simulink library "hdlsllibUNLOCKED"  (R2019a)
settings: Solver=ode45  StartTime=0.0  StopTime=10.0  RelTol=1e-3  EnableMultiTasking=on
values from neighbouring files (symbols this model uses):
  freerun = strcmp(get_param(blk, 'CountType'), 'Free running')    [hdlblkmask_counter.m]
  maxval_sc = countrange(2)    [hdlblkmask_counter.m]
  samptime = -1    [hdlblkmask_counter.m]
undefined symbols (not defined in the file or in its folder): a, b, c, Dialog, DiscIntNeverNeededParam, Floor, HDLStatusEnum, jsin, magnitude, message, Newton, NumBits1, NumBits2, Raphson, Slope1, Slope2
libraries: simulink x70, $bdroot x5, hdlmdlgenlib x1, hdlsllib_helper x1
(part 1 of 3)
settings Model: Creator=The MathWorks, Inc kinda  LastModifiedBy=Bailey
settings DataIOCC: LimitDataPoints=on  SaveFormat=Array  ReturnWorkspaceOutputs=off
settings OptimizationCC: LifeSpan=inf
settings DebuggingCC: UnderspecifiedInitializationDetection=Classic  MergeDetectMultiDrivingBlocksExec=none  SolverPrmCheckMsg=warning  AllowSymbolicDim=off  PregeneratedLibrarySubsystemCodeDiagnostic=none  SFUnexpectedBacktrackingDiag=warning  SFNoUnconditionalDefaultTransitionDiag=warning  SFExecutionAtInitializationDiag=none  ArithmeticOperatorsInVariantConditions=warning
settings HardwareCC: ProdBitPerPointer=32  ProdBitPerSizeT=32  ProdBitPerPtrDiffT=32  ProdLargestAtomicFloat=None  ProdIntDivRoundTo=Undefined  ProdEndianess=Unspecified  ProdWordSize=32  ProdHWDeviceType=32-bit Generic
settings ModelReferenceCC: PropagateSignalLabelsOutOfModel=off
settings SFSimCC: SimUseLocalCustomCode=off
settings RTWCC: RTWUseLocalCustomCode=off
settings CodeAppCC: StateflowObjectComments=on
settings GRTTargetCC: TargetLangStandard=C89/C90 (ANSI)  GeneratePreprocessorConditionals=Disable all
settings ConfigComp: CovScope=ReferencedModels  CovMetricSettings=dw  CovHtmlReporting=on  CovSaveCumulativeToWorkspaceVar=on  CovSaveSingleToWorkspaceVar=on  CovShowResultsExplorer=off  CovExternalEMLEnable=off  CovSFcnEnable=off

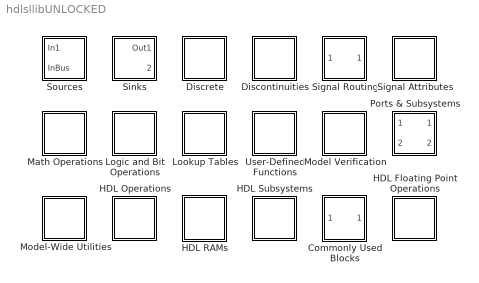
== system hdlsllibUNLOCKED ==
  Commonly Used Blocks : Subsystem
      mask Display: image('commonly_used.bmp')
  Discontinuities : Subsystem
      mask Display: image('nonlinear.bmp')
  Discrete : Subsystem
      mask Display: image('discrete.bmp')
  HDL Subsystems : Subsystem
      mask Display:
      | image('blank_block.bmp')
      | color('darkBlue')
      | fprintf('HDL\nSubsys\n')
  HDL Floating Point Operations : Subsystem
      mask Display:
      | image('blank_block.bmp')
      | color('darkBlue')
      | fprintf(' HDL\nNFP')
  HDL Operations : Subsystem
      mask Display:
      | image('blank_block.bmp')
      | color('darkBlue')
      | fprintf(' HDL\nOPS')
  HDL RAMs : Subsystem
      mask Display:
      | image('blank_block.bmp')
      | color('darkBlue')
      | fprintf(' HDL\nRAMs')
  Logic and Bit Operations : Subsystem
      mask Display: image('logical_bit.bmp')
  Lookup Tables : Subsystem
      mask Display: image('tables.bmp')
  Math Operations : Subsystem
      mask Display: image('math.bmp')
  Model Verification : Subsystem
      mask Display: image('assertion.bmp')
  Model-Wide Utilities : Subsystem
      mask Display:
      | image('blank_block.bmp')
      | color('darkBlue')
      | disp('Misc')
  Ports & Subsystems : Subsystem
      settings: CopyFcn=set_param(gcbh,'LinkStatus','none'); set_param(gcbh,'Mask','off'); set_param(gcbh,'MaskType',''); set_param(gcbh,'MaskDescription',''); set_param(gcbh,'OpenFcn',''); set_param(gcbh,'CopyFcn','')
      mask Display: image('subsystems.bmp')
  Signal Attributes : Subsystem
      mask Display: image('attributes.bmp')
  Signal Routing : Subsystem
      mask Display: image('signals.bmp')
  Sinks : Subsystem
      mask Display: image('sinks.bmp')
  Sources : Subsystem
      mask Display: image('sources.bmp')
  User-Defined Functions : Subsystem
      mask Display: image('functions.bmp')

== system hdlsllibUNLOCKED/Commonly Used Blocks ==
  In1 : Inport
  Constant : Constant
  Data Type Conversion : DataTypeConversion
  Delay : Delay  DelayLength=1  InitialCondition=0
  Demux : Demux  Outputs=2
  Gain : Gain
  Logical Operator : Logic  AllPortsSameDT=off  OutDataTypeStr=boolean
  Mux : Mux  Inputs=2
  Product : Product
  Relational Operator : RelationalOperator  Operator=<=  OutDataTypeStr=boolean  RndMeth=Nearest
  Scope : Scope
  Sum : Sum  Inputs=|++
  Switch : Switch
  Out1 : Outport

== system hdlsllibUNLOCKED/Discontinuities ==
  Backlash : Backlash
  Coulomb & Viscous Friction : simulink/Discontinuities/Coulomb & Viscous Friction  offset=[1 3 2 0]  gain=1
      settings: SourceProductName=Simulink
  Dead Zone : DeadZone  SaturateOnIntegerOverflow=on
  Dead Zone Dynamic : simulink/Discontinuities/Dead Zone Dynamic
      settings: SourceProductName=Simulink  SourceProductBaseCode=SL
  Hit Crossing : HitCross  HitCrossingDirection=rising
  Relay : Relay
  Saturation : Saturate
  Saturation Dynamic : simulink/Discontinuities/Saturation Dynamic  OutMin=[]  OutMax=[]  OutDataTypeStr=Inherit: Same as second input  OutDataType=fixdt(1, 16)  OutScaling=2^-10  DoSatur=off
  Wrap To Zero : simulink/Discontinuities/Wrap To Zero  Threshold=255
      settings: SourceProductName=Simulink  SourceProductBaseCode=SL

== system hdlsllibUNLOCKED/Discrete ==
  Delay : Delay
  Discrete Transfer Fcn : DiscreteTransferFcn
  Discrete FIR Filter : DiscreteFir
  Discrete PID Controller : simulink/Continuous/PID Controller  Controller=PID  Form=Parallel  TimeDomain=Discrete-time  SampleTime=-1  IntegratorMethod=Forward Euler  FilterMethod=Forward Euler  ControllerParametersSource=internal  P=1  I=1  D=0  UseFilter=on  N=100  TunerSelectOption=Transfer Function Based (PID Tuner App)  InitialConditionSource=internal  InitialConditionForIntegrator=0  InitialConditionForFilter=0  DifferentiatorICPrevScaledInput=0  ExternalReset=none  TrackingMode=off  Kt=1  LimitOutput=off  UpperSaturationLimit=inf  LowerSaturationLimit=-inf  LinearizeAsGain=off  AntiWindupMode=none  Kb=1  POutMin=[]  POutMax=[]  IOutMin=[]  IOutMax=[]  DOutMin=[]  DOutMax=[]  NOutMin=[]  NOutMax=[]  SumOutMin=[]  SumOutMax=[]  SaturationOutMin=[]  SaturationOutMax=[]  PParamMin=[]  PParamMax=[]  IParamMin=[]  IParamMax=[]  DParamMin=[]  DParamMax=[]  NParamMin=[]  NParamMax=[]  KbParamMin=[]  KbParamMax=[]  KtParamMin=[]  KtParamMax=[]  KbOutMin=[]  KbOutMax=[]  KtOutMin=[]  KtOutMax=[]  IntegratorOutMin=[]  IntegratorOutMax=[]  FilterOutMin=[]  FilterOutMax=[]  SumI1OutMin=[]  SumI1OutMax=[]  SumI2OutMin=[]  SumI2OutMax=[]  SumI3OutMin=[]  SumI3OutMax=[]  SumI4OutMin=[]  SumI4OutMax=[]  SumDOutMin=[]  SumDOutMax=[]  DifferentiatorOutMin=[]  DifferentiatorOutMax=[]  FilterDiffOutCoefMin=[]  FilterDiffOutCoefMax=[]  ReciprocalOutMin=[]  ReciprocalOutMax=[]  SumDenOutMin=[]  SumDenOutMax=[]  SumNumOutMin=[]  SumNumOutMax=[]  DivideOutMin=[]  DivideOutMax=[]  IntegratorContinuousStateAttributes=''  IntegratorStateMustResolveToSignalObject=off  IntegratorRTWStateStorageClass=Auto  FilterContinuousStateAttributes=''  FilterStateMustResolveToSignalObject=off  FilterRTWStateStorageClass=Auto  ParallelPVariant=InternalParameters  IdealPVariant=Disabled  IVariant=InternalParameters  DVariant=InternalParameters  IntegratorVariant=Discrete  SatVariant=Disabled  AWVariant=Passthrough  PCopyVariant=Disabled  TRVariant=Disabled  FdbkBlocksVariant=Forward  IdealPFdbkVariant=Disabled  SatFdbkVariant=Disabled  DerivativeFilterVariant=ForwardEulerFilter  NVariant=InternalParameters  NCopyVariant=Disabled  FilterICVariant=InternalICsFilter  IntegratorICVariant=InternalICs  ExternalResetVariant=Disabled  TRSumVariant=Passthrough  SumFdbkVariant=Disabled  SumVariant=Sum_PID
  Discrete-Time Integrator : DiscreteIntegrator  SampleTime=-1  ICPrevOutput=DiscIntNeverNeededParam  ICPrevScaledInput=DiscIntNeverNeededParam
  Enabled Delay : Delay  ShowEnablePort=on
      settings: InputPortMap=u0,e6
  Enabled Resettable Delay : Delay  DelayLength=1  ExternalReset=Level  ShowEnablePort=on
      settings: InputPortMap=u0,e6,r5
  Memory : Memory  InheritSampleTime=on
  Resettable Delay : Delay  DelayLength=1  ExternalReset=Level
      settings: InputPortMap=u0,r5
  Tapped Delay : simulink/Discrete/Tapped Delay  vinit=0.0  samptime=-1  NumDelays=4  DelayOrder=Oldest  includeCurrent=off
  Unit Delay : UnitDelay  SampleTime=-1  HasFrameUpgradeWarning=on
  Unit Delay Enabled Synchronous : Subsystem  mask(Unit Delay Enabled Synchronous){InitialCondition=0.0, SampleTime=-1}
      mask prompts: InitialCondition "Simulink:blkprm_prompts:DelayBlkInitCond"; SampleTime "Simulink:blkprm_prompts:AllBlksSampleTime"
      mask help:
      | Normally, the output is the signal u delayed by one sample period.
      | When the enable signal is false, the block is disabled, and the state and output values do not change. The enable action only supports scalar inputs. Scalar expansion is used for the enable action when the signal u is a vector.
      mask Help: helpview([docroot '/simulink/helptargets.map'],'HDL_Unit_Delay_Enabled_Synchronous');
      mask TypeOptions InitialCondition: Unit Delay Enabled/Enabled Delay/InitialCondition
      mask TypeOptions SampleTime: Unit Delay Enabled/Enabled Delay/SampleTime
      mask DialogControl InitialCondition Prompt: Initial condition:
      mask DialogControl SampleTime Prompt: Sample time (-1 for inherited):
      mask Display: dpoly([0 1],[1 0],'z');
  Unit Delay Enabled Resettable Synchronous : Subsystem  mask(Unit Delay Enabled Resettable Synchronous){InitialCondition=0.0, SampleTime=-1}
      mask prompts: InitialCondition "Simulink:blkprm_prompts:DelayBlkInitCond"; SampleTime "Simulink:blkprm_prompts:AllBlksSampleTime"
      mask help:
      | Normally, the output is the signal u delayed by one sample period.
      | When the enable signal is false, the block is disabled, and the state and output values do not change. The enable action only supports scalar inputs. Scalar expansion is used for the enable action when the signal u is a vector.
      | When the reset signal R is true, the state and the output are always set equal to the initial condition parameter. This block exhibits hardware-friendly reset behavior. This reset action only supports scalar inputs. Scalar expansion is used for this reset action when the signal u is a vector.
      mask Help: helpview([docroot '/simulink/helptargets.map'],'HDL_Unit_Delay_Enabled_Resettable_Synchronous');
      mask TypeOptions InitialCondition: Unit Delay Enabled Resettable/Enabled Resettable Delay/InitialCondition
      mask TypeOptions SampleTime: Unit Delay Enabled Resettable/Enabled Resettable Delay/SampleTime
      mask DialogControl InitialCondition Prompt: Initial condition:
      mask DialogControl SampleTime Prompt: Sample time (-1 for inherited):
      mask Display: dpoly([0 1],[1 0],'z');
  Unit Delay Resettable Synchronous : Subsystem  mask(Unit Delay Resettable Synchronous){InitialCondition=0.0, SampleTime=-1}
      mask prompts: InitialCondition "Simulink:blkprm_prompts:DelayBlkInitCond"; SampleTime "Simulink:blkprm_prompts:AllBlksSampleTime"
      mask help:
      | Normally, the output is the signal u delayed by one sample period.
      | When the reset signal R is true, the state and the output are always set equal to the initial condition parameter. This block exhibits hardware-friendly reset behavior. This reset action only supports scalar inputs. Scalar expansion is used for this reset action when the signal u is a vector.
      mask Help: helpview([docroot '/simulink/helptargets.map'],'HDL_Unit_Delay_Resettable_Synchronous');
      mask TypeOptions InitialCondition: Unit Delay Resettable/Resettable Delay/InitialCondition
      mask TypeOptions SampleTime: Unit Delay Resettable/Resettable Delay/SampleTime
      mask DialogControl InitialCondition Prompt: Initial condition:
      mask DialogControl SampleTime Prompt: Sample time (-1 for inherited):
      mask Display: dpoly([0 1],[1 0],'z');
  Zero-Order Hold : ZeroOrderHold  SampleTime=-1

== system hdlsllibUNLOCKED/HDL Subsystems ==
  Enabled Synchronous Subsystem : Subsystem  TreatAsAtomicUnit=on  mask(Enabled Synchronous Subsystem){}
      mask help: Simulink:masks:EnabledSynchronousSubsystem_MP
      settings: CopyFcn=set_param(gcbh,'LinkStatus','none'); set_param(gcbh,'Mask','off'); set_param(gcbh,'MaskType',''); set_param(gcbh,'MaskDescription',''); set_param(gcbh,'OpenFcn',''); set_param(gcbh,'CopyFcn','')  OpenFcn=open_system(gcbh,'force')
  Resettable Synchronous Subsystem : Subsystem  TreatAsAtomicUnit=on  mask(Resettable Synchronous Subsystem){}
      mask help: Simulink:masks:ResettableSynchronousSubsystem_MP
      settings: CopyFcn=set_param(gcbh,'LinkStatus','none'); set_param(gcbh,'Mask','off'); set_param(gcbh,'MaskType',''); set_param(gcbh,'MaskDescription',''); set_param(gcbh,'OpenFcn',''); set_param(gcbh,'CopyFcn','')  OpenFcn=open_system(gcbh,'force')
  State Control : StateControl  StateControl=Synchronous
  Synchronous Subsystem : Subsystem  mask(Synchronous Subsystem){}
      mask help: Simulink:masks:SynchronousSubsystem_MP
      settings: CopyFcn=set_param(gcbh,'LinkStatus','none'); set_param(gcbh,'Mask','off'); set_param(gcbh,'MaskType',''); set_param(gcbh,'MaskDescription',''); set_param(gcbh,'OpenFcn',''); set_param(gcbh,'CopyFcn','')  OpenFcn=open_system(gcbh,'force')

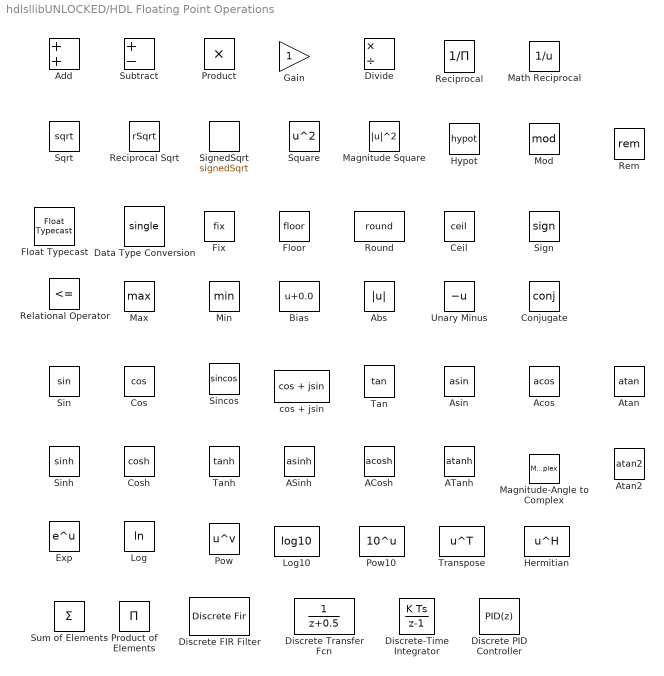
== system hdlsllibUNLOCKED/HDL Floating Point Operations ==
  ACosh : Trigonometry  Operator=acosh
  ASinh : Trigonometry  Operator=asinh
  ATanh : Trigonometry  Operator=atanh
  Abs : Abs
  Acos : Trigonometry  Operator=acos
  Add : Sum
  Asin : Trigonometry  Operator=asin
  Atan : Trigonometry  Operator=atan
  Atan2 : Trigonometry  Operator=atan2
  Bias : Bias  Bias=0.0
  Ceil : Rounding  Operator=ceil
  Conjugate : Math  Operator=conj  RndMeth=Zero  SaturateOnIntegerOverflow=on
  Cos : Trigonometry  Operator=cos
  Cosh : Trigonometry  Operator=cosh
  Data Type Conversion : DataTypeConversion  OutDataTypeStr=single  RndMeth=Nearest
  Discrete Transfer Fcn : DiscreteTransferFcn
  Discrete FIR Filter : DiscreteFir
  Discrete PID Controller : simulink/Continuous/PID Controller  Controller=PID  Form=Parallel  TimeDomain=Discrete-time  SampleTime=-1  IntegratorMethod=Forward Euler  FilterMethod=Forward Euler  ControllerParametersSource=internal  P=1  I=1  D=0  UseFilter=on  N=100  TunerSelectOption=Transfer Function Based (PID Tuner App)  InitialConditionSource=internal  InitialConditionForIntegrator=0  InitialConditionForFilter=0  DifferentiatorICPrevScaledInput=0  ExternalReset=none  TrackingMode=off  Kt=1  LimitOutput=off  UpperSaturationLimit=inf  LowerSaturationLimit=-inf  LinearizeAsGain=off  AntiWindupMode=none  Kb=1  POutMin=[]  POutMax=[]  IOutMin=[]  IOutMax=[]  DOutMin=[]  DOutMax=[]  NOutMin=[]  NOutMax=[]  SumOutMin=[]  SumOutMax=[]  SaturationOutMin=[]  SaturationOutMax=[]  PParamMin=[]  PParamMax=[]  IParamMin=[]  IParamMax=[]  DParamMin=[]  DParamMax=[]  NParamMin=[]  NParamMax=[]  KbParamMin=[]  KbParamMax=[]  KtParamMin=[]  KtParamMax=[]  KbOutMin=[]  KbOutMax=[]  KtOutMin=[]  KtOutMax=[]  IntegratorOutMin=[]  IntegratorOutMax=[]  FilterOutMin=[]  FilterOutMax=[]  SumI1OutMin=[]  SumI1OutMax=[]  SumI2OutMin=[]  SumI2OutMax=[]  SumI3OutMin=[]  SumI3OutMax=[]  SumI4OutMin=[]  SumI4OutMax=[]  SumDOutMin=[]  SumDOutMax=[]  DifferentiatorOutMin=[]  DifferentiatorOutMax=[]  FilterDiffOutCoefMin=[]  FilterDiffOutCoefMax=[]  ReciprocalOutMin=[]  ReciprocalOutMax=[]  SumDenOutMin=[]  SumDenOutMax=[]  SumNumOutMin=[]  SumNumOutMax=[]  DivideOutMin=[]  DivideOutMax=[]  IntegratorContinuousStateAttributes=''  IntegratorStateMustResolveToSignalObject=off  IntegratorRTWStateStorageClass=Auto  FilterContinuousStateAttributes=''  FilterStateMustResolveToSignalObject=off  FilterRTWStateStorageClass=Auto  ParallelPVariant=InternalParameters  IdealPVariant=Disabled  IVariant=InternalParameters  DVariant=InternalParameters  IntegratorVariant=Discrete  SatVariant=Disabled  AWVariant=Passthrough  PCopyVariant=Disabled  TRVariant=Disabled  FdbkBlocksVariant=Forward  IdealPFdbkVariant=Disabled  SatFdbkVariant=Disabled  DerivativeFilterVariant=ForwardEulerFilter  NVariant=InternalParameters  NCopyVariant=Disabled  FilterICVariant=InternalICsFilter  IntegratorICVariant=InternalICs  ExternalResetVariant=Disabled  TRSumVariant=Passthrough  SumFdbkVariant=Disabled  SumVariant=Sum_PID
  Discrete-Time Integrator : DiscreteIntegrator  SampleTime=-1  ICPrevOutput=DiscIntNeverNeededParam  ICPrevScaledInput=DiscIntNeverNeededParam
  Divide : Product  Inputs=*/
  Exp : Math  SaturateOnIntegerOverflow=on
  Fix : Rounding  Operator=fix
  Float Typecast : FloatTypecast
  Floor : Rounding
  Gain : Gain
  Hermitian : Math  Operator=hermitian  RndMeth=Zero  SaturateOnIntegerOverflow=on
  Hypot : Math  Operator=hypot  RndMeth=Zero  SaturateOnIntegerOverflow=on
  Log : Math  Operator=log  SaturateOnIntegerOverflow=on
  Log10 : Math  Operator=log10  RndMeth=Zero  SaturateOnIntegerOverflow=on
  Magnitude Square : Math  Operator=magnitude^2  RndMeth=Zero  SaturateOnIntegerOverflow=on
  Magnitude-Angle to Complex : MagnitudeAngleToComplex
  Math Reciprocal : Math  Operator=reciprocal  SaturateOnIntegerOverflow=on
  Max : MinMax  Function=max
  Min : MinMax
  Mod : Math  Operator=mod  SaturateOnIntegerOverflow=on
  Pow : Math  Operator=pow  RndMeth=Zero  SaturateOnIntegerOverflow=on
  Pow10 : Math  Operator=10^u  RndMeth=Zero  SaturateOnIntegerOverflow=on
  Product : Product
  Product of Elements : Product  Inputs=*
  Reciprocal : Product  Inputs=/  SaturateOnIntegerOverflow=on  RndMeth=Zero
  Reciprocal Sqrt : Sqrt  Operator=rSqrt  IntermediateResultsDataTypeStr=double  SaturateOnIntegerOverflow=on
  Relational Operator : RelationalOperator  Operator=<=  OutDataTypeStr=boolean  RndMeth=Simplest
  Rem : Math  Operator=rem  SaturateOnIntegerOverflow=on
  Round : Rounding  Operator=round
  Sign : Signum
  SignedSqrt : Sqrt  Operator=signedSqrt  IntermediateResultsDataTypeStr=single  SaturateOnIntegerOverflow=on
  Sin : Trigonometry
  Sincos : Trigonometry  Operator=sincos
  Sinh : Trigonometry  Operator=sinh
  Sqrt : Sqrt  IntermediateResultsDataTypeStr=double  SaturateOnIntegerOverflow=on
  Square : Math  Operator=square  RndMeth=Zero  SaturateOnIntegerOverflow=on
  Subtract : Sum  Inputs=+-
  Sum of Elements : Sum  Inputs=+
  Tan : Trigonometry  Operator=tan
  Tanh : Trigonometry  Operator=tanh
  Transpose : Math  Operator=transpose  RndMeth=Zero  SaturateOnIntegerOverflow=on
  Unary Minus : UnaryMinus
  cos + jsin : Trigonometry  Operator=cos + jsin

== system hdlsllibUNLOCKED/HDL Operations ==
  Deserializer1D : Subsystem  mask(Deserializer1D){Ratio=1, IdleCycles=0, InitialCondition=0, startIn=off, validIn=off, validOut=off, inputDataDimensions=-1, inputSampleTime=-1, inputSignalType=auto}
      mask prompts: Ratio "Ratio (Output Vector Size/Input Vector Size)"; IdleCycles "Idle Cycles"; InitialCondition "Initial condition"; inputDataDimensions "Input data port dimensions (-1 for inherited)"; inputSampleTime "Input sample time (-1 for inherited)"; inputSignalType "Input signal type"
      mask help: Convert from scalar to vector, or from smaller-size vector to larger-size vector. The output rate is S / (Ratio + Idle Cycles), where S is the input rate.
      mask init:
      | hdlblkmask_deserializer1D.mask_init(gcb);
      settings: MinAlgLoopOccurrences=on
      mask Help: helpview([docroot '/simulink/helptargets.map'],'HDL_deserializer1D');
      mask TypeOptions Ratio: HDL1DDs/Ratio
      mask Callback Ratio: hdlblkmask_deserializer1D.ratio_callback(gcb);
      mask TypeOptions IdleCycles: HDL1DDs/IdleCycles
      mask Callback IdleCycles: hdlblkmask_deserializer1D.ratio_callback(gcb);
      mask Callback InitialCondition: hdlblkmask_deserializer1D.initialCondition_callback(gcb);
      mask TypeOptions startIn: HDL1DDs/StartInPortEnb
      mask TypeOptions validIn: HDL1DDs/ValidInPortEnb
      mask Callback inputDataDimensions: hdlblkmask_deserializer1D.InDataDimensions_callback(gcb);
      mask Callback inputSampleTime: hdlblkmask_deserializer1D.InSampleTime_callback(gcb);
      mask TypeOptions inputSignalType: auto | real | complex
      mask Callback inputSignalType: hdlblkmask_deserializer1D.InSignalType_callback(gcb);
      mask DialogControl Container7 Prompt: Main
      mask DialogControl ControlPorts Prompt: Control Signal Ports
      mask DialogControl Container10 Prompt: Signal Attributes
  Multiply-Accumulate : Subsystem  mask(Multiply-Accumulate){opMode=Vector, initValueSetting=Dialog, initValue=0, initValueSetting2=Dialog, initValue2=0, initValueSetting3=Dialog, initValue3=0, num_samples=2, RndMeth=Floor, RndMeth2=Floor, RndMeth3=Floor, OutDataTypeStr=Inherit: Inherit via internal rule, datatype2=Inherit: Inherit via back propagation, datatype3=Inherit: Inherit via back propagation, validOut=on, endInandOut=on, startOut=on, countOut=on, dim=-1, DoSatur=off, parallel=off}
      mask prompts: opMode "Operation Mode:"; num_samples "Number of Samples:"; RndMeth "Integer rounding mode:"; RndMeth2 "Integer rounding mode:"; RndMeth3 "Integer rounding mode:"; OutDataTypeStr "Simulink:blkprm_prompts:OUTPUT_UNIFIEDDATATYPE"; datatype2 "Output data type"; datatype3 "Output data type:"; validOut "Enable valid output port"; endInandOut "Enable end input and output ports"; startOut "Enable start output port"; countOut "Enable count output port"; dim "Specify input dimensions [M,N]"; DoSatur "Simulink:blkprm_prompts:AllBlksSaturate"; parallel "Use fully parallel implementation"
      mask help:
      | Operation Mode: Vector
      | 	dataOut= sum(a.*b) + c
      |
      | Operation Mode: Streaming- using Start and End ports
      | 	dataOut(t+1)= dataOut(t) + sum(a(t)*b(t)) + c
      | 	where c=bias when start and valid=high,
      | 	else c=0
      |
      | Operation Mode: Streaming- using number of Samples
      | 	dataOut(t+1)= dataOut(t) + sum(a(t)*b(t)) + c
      | 	where c=bias when t=0
      | 	else c=0
      |
      | This block is designed for efficient mapping to DSP slices on FPGAs.
      mask init:
      | hdlblkmask_multiplyAccumulate(gcb)
      mask TypeOptions opMode: Vector | Streaming - using Start and End ports | Streaming - using Number of Samples
      mask Callback opMode: hdlblkmask_multiplyAccumulate_cb1(gcb)
      mask TypeOptions initValueSetting: vectorMAC/initValueSetting
      mask Callback initValueSetting: hdlblkmask_multiplyAccumulate_cb.input_bias_cb1(gcb)
      mask TypeOptions initValue: vectorMAC/initValue
      mask TypeOptions initValueSetting2: streamingMAC_without_counter/initValueSetting
      mask Callback initValueSetting2: hdlblkmask_multiplyAccumulate_cb.input_bias_cb2(gcb)
      mask TypeOptions initValue2: streamingMAC_without_counter/initValue
      mask TypeOptions initValueSetting3: streamingMAC_with_counter/initValueSetting
      mask Callback initValueSetting3: hdlblkmask_multiplyAccumulate_cb.input_bias_cb3(gcb)
      mask TypeOptions initValue3: streamingMAC_with_counter/initValue
      mask TypeOptions num_samples: streamingMAC_with_counter/num_samples
      mask Callback num_samples: hdlblkmask_streaming_number_of_samples_cb(gcb);
      mask TypeOptions RndMeth: vectorMAC/RndMeth
      mask TypeOptions RndMeth2: streamingMAC_without_counter/RndMeth
      mask TypeOptions RndMeth3: streamingMAC_with_counter/RndMeth
      mask TypeOptions OutDataTypeStr: vectorMAC/AccumDataTypeStr
      mask TypeOptions datatype2: streamingMAC_without_counter/typeinfo
      mask TypeOptions datatype3: streamingMAC_with_counter/typeinfo
      mask TypeOptions DoSatur: vectorMAC/DoSatur
      mask DialogControl Container7 Prompt: Data
      mask DialogControl biastxt1 Prompt: Bias:
      mask DialogControl biastxt2 Prompt: Bias:
      mask DialogControl biastxt3 Prompt: Bias:
      mask DialogControl OutDataTypeStr Prompt: Output data type:
      mask DialogControl ports_container Prompt: Ports
      mask DialogControl DoSatur Prompt: Saturate on integer overflow
      mask Display:
      | opMode = get_param(gcb,'opMode');
      | maskVal = get_param(gcb,'MaskValues');
      | switch opMode
      |     case 'Vector'
      |         setting = maskVal{2};
      |     case 'Streaming - using Start and End ports'
      |         setting = maskVal{4};
      | 
      |     case 'Streaming - using Number of Samples'
      |         setting = maskVal{6};
      | end
      | 
      | if(strcmp(setting,'Input port'))
      |     disp([char(8721),'a(i)*b(i)+c'])
      | else
      |     disp([char(8721),'a(i)*b(i)'])
      | end
  Multiply-Add : Subsystem  mask(Multiply-Add){Function=c+(a.*b), datatype=Inherit: Inherit via internal rule, RndMeth=Floor, DoSatur=off, FMA=off}
      mask prompts: datatype "Output data type"; RndMeth "Integer rounding mode"; DoSatur "Saturate on integer overflow"; FMA "Floating-point fused multiply-add (FMA)"
      mask help: Multiply first two inputs and add result to third input or subtract result from third input. The function option defines the mode of operation. This block is designed for efficient mapping to DSP slices on FPGAs.
      mask init:
      | hdlblkmask_multiplyadd
      mask Help: helpview([docroot '/simulink/helptargets.map'],'HDL_Multiply_Add');
      mask TypeOptions Function: c+(a.*b) | c-(a.*b) | (a.*b)-c
      mask TypeOptions RndMeth: Ceiling | Convergent | Floor | Nearest | Round | Simplest | Zero
      mask Callback RndMeth: hdlblkmask_multiplyadd
      mask Display:
      | port_label('input', 1, 'a');
      | port_label('input', 2, 'b');
      | port_label('input', 3, 'c');
      | disp(get_param(gcb,'Function'));
  Serializer1D : Subsystem  mask(Serializer1D){Ratio=1, IdleCycles=0, validIn=off, startOut=off, validOut=off, inputDataDimensions=-1, inputSampleTime=-1, inputSignalType=auto}
      mask prompts: Ratio "Ratio (Input Vector Size/Output Vector Size)"; IdleCycles "Idle Cycles"; inputDataDimensions "Input data port dimensions (-1 for inherited)"; inputSampleTime "Input sample time (-1 for inherited)"; inputSignalType "Input signal type"
      mask help: Convert from vector to scalar, or to smaller-size vector. The output rate is V * (Ratio + Idle Cycles), where V is the input rate.
      mask init:
      | hdlblkmask_serializer1D.mask_init(gcb);
      mask Help: helpview([docroot '/simulink/helptargets.map'],'HDL_serializer1D');
      mask TypeOptions Ratio: HDL1DSe/Ratio
      mask Callback Ratio: hdlblkmask_serializer1D.ratio_callback(gcb);
      mask TypeOptions IdleCycles: HDL1DSe/IdleCycles
      mask Callback IdleCycles: hdlblkmask_serializer1D.ratio_callback(gcb);
      mask Callback inputDataDimensions: hdlblkmask_serializer1D.InDataDimensions_callback(gcb);
      mask Callback inputSampleTime: hdlblkmask_serializer1D.InSampleTime_callback(gcb);
      mask TypeOptions inputSignalType: auto | real | complex
      mask Callback inputSignalType: hdlblkmask_serializer1D.InSignalType_callback(gcb);
      mask DialogControl Container9 Prompt: Main
      mask DialogControl ControlPorts Prompt: Control Signal Ports
      mask DialogControl Container10 Prompt: Signal Attributes

== system hdlsllibUNLOCKED/HDL RAMs ==
  Dual Port RAM : Subsystem  mask(Dual-port RAM){ram_size=8}
      mask prompts: ram_size "Address port width (2 to 29 bits)"
      mask help: This block simulates a dual-port RAM with two data output ports.
      mask init:
      | hdlblkmask_dpram;
      mask Help: helpview([docroot '/simulink/helptargets.map'],'HDL_dual_port_RAM');
  Dual Port RAM System : MATLABSystem  System=hdl.RAM  RAMType=Dual port  WriteOutputValue=New data  RAMInitialValue=0  SimulateUsing=Code generation
      mask Type: hdl.RAM
      mask Display:
      | disp(['Dual Port' char(10) 'RAM']);
      | port_label('input',1,'din');
      | port_label('input',2,'wr_addr');
      | port_label('input',3,'wr_en');
      | port_label('input',4,'rd_addr');
      | port_label('output',1,'wr_dout');
      | port_label('output',2,'rd_dout');
  Dual Rate Dual Port RAM : Subsystem  mask(Dual-rate dual-port RAM){ram_size=8}
      mask prompts: ram_size "Address port width (2 to 28 bits)"
      mask help: This block simulates a dual-clock dual-port RAM with two data output ports.
      mask init:
      | hdlblkmask_drdpram();
      mask Help: helpview([docroot '/simulink/helptargets.map'],'HDL_dual_rate_dual_port_ram');
  HDL FIFO : Subsystem  mask(HDL_FIFO){fifo_size=10, ratio=1, push_msg=Warning, pop_msg=Warning, show_empty=on, show_full=on, show_num=on}
      mask prompts: fifo_size "Register size:"; ratio "The ratio of output sample time to input sample time: <br>(Must be either a positive integer or 1/N, where N is a positive integer)"; push_msg "Push onto full register:"; pop_msg "Pop empty register:"; show_empty "Show empty register indicator port (Empty)"; show_full "Show full register indicator port (Full)"; show_num "Show number of register entries port (Num)"
      mask help: Implements a synchronous "First In, First Out" (FIFO) register.
      mask init:
      | hdlblkmask_fifo('init');
      settings: ErrorFcn=hdlblkmask_fifo_updatemsg
      mask Help: helpview([docroot '/simulink/helptargets.map'],'HDL_FIFO');
      mask Callback fifo_size: hdlblkmask_fifo('size_check')
      mask Callback ratio: hdlblkmask_fifo('ratio_check')
      mask TypeOptions push_msg: Ignore | Warning | Error
      mask TypeOptions pop_msg: Ignore | Warning | Error
  Simple Dual Port RAM System : MATLABSystem  System=hdl.RAM  RAMType=Simple dual port  WriteOutputValue=New data  RAMInitialValue=0  SimulateUsing=Code generation
      mask Type: hdl.RAM
      mask Display:
      | disp(['Simple' char(10) 'Dual Port' char(10) 'RAM']);
      | port_label('input',1,'din');
      | port_label('input',2,'wr_addr');
      | port_label('input',3,'wr_en');
      | port_label('input',4,'rd_addr');
      | port_label('output',1,'rd_dout');
  Simple Dual Port RAM : Subsystem  mask(Simple Dual-port RAM){ram_size=8}
      mask prompts: ram_size "Address port width (2 to 29 bits)"
      mask help: This block simulates a simple dual-port RAM with one data output port.
      mask init:
      | hdlblkmask_dpram;
      mask Help: helpview([docroot '/simulink/helptargets.map'],'HDL_simple_dual_port_ram');
  Single Port RAM : Subsystem  mask(Single-port RAM){ram_size=8, dout_type=New data}
      mask prompts: ram_size "Address port width (2 to 29 bits)"; dout_type "Output data during write:"
      mask help: This block simulates a single-port RAM.
      mask init:
      | hdlblkmask_dpram;
      mask Help: helpview([docroot '/simulink/helptargets.map'],'HDL_single_port_ram');
      mask TypeOptions dout_type: New data | Old data
  Single Port RAM System : MATLABSystem  System=hdl.RAM  RAMType=Single port  WriteOutputValue=New data  RAMInitialValue=0  SimulateUsing=Code generation
      mask Type: hdl.RAM
      mask Display:
      | disp(['Single Port' char(10) 'RAM']);
      | port_label('input',1,'din');
      | port_label('input',2,'addr');
      | port_label('input',3,'wr_en');
      | port_label('output',1,'dout');

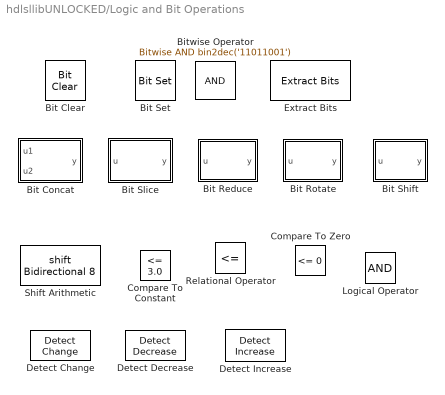
== system hdlsllibUNLOCKED/Logic and Bit Operations ==
  Bit Clear : simulink/Logic and Bit Operations/Bit Clear  iBit=0
      settings: SourceProductName=Simulink  SourceProductBaseCode=SL
  Bit Concat : Subsystem  TreatAsAtomicUnit=on  mask(Bit Concat){numInputs=2}
      mask prompts: numInputs "Number of Inputs"
      mask help: Concatenate the input words. For scalar inputs, two or more input signals should be connected to the block. For vector inputs, at least one input should be connected to the block. The left-right ordering of words in the output follows the ordering of input signals. The L input is the lowest-order word and the H input is the highest order word.
      mask init:
      | [blkname, portLabels] = hdlblkmask_bitconcat_eml;
      mask Help: helpview([docroot '/simulink/helptargets.map'],'HDL_bit_concat');
      mask Display:
      | disp(blkname);
      | port_label('input',portLabels(1).port,portLabels(1).txt);
      | port_label('input',portLabels(2).port,portLabels(2).txt);
  Bit Reduce : Subsystem  TreatAsAtomicUnit=on  mask(Bit Reduce){mode=AND}
      mask prompts: mode "Reduction Mode"
      mask help: Perform a bitwise AND, OR, or XOR reduction of the input signal, as specified by the Reduction Mode parameter.
      mask init:
      | blkname = hdlblkmask_bitreduce;
      mask Help: helpview([docroot '/simulink/helptargets.map'],'HDL_bit_reduce');
      mask TypeOptions mode: AND | OR | XOR
      mask Display: disp(blkname);
  Bit Rotate : Subsystem  TreatAsAtomicUnit=on  mask(Bit Rotate){mode=Rotate Left, N=0}
      mask prompts: mode "Rotate Mode"; N "Rotate Length (must be greater than or equal to zero)"
      mask help: Rotate the input signal left or right as specified by the Rotate Mode parameter. The Rotate Length specifies the number of bits to be rotated.
      mask init:
      | blkname = hdlblkmask_bitrotate;
      mask Help: helpview([docroot '/simulink/helptargets.map'],'HDL_bit_rotate');
      mask TypeOptions mode: Rotate Left | Rotate Right
      mask Display: disp(blkname);
  Bit Set : simulink/Logic and Bit Operations/Bit Set  iBit=0
      settings: SourceProductName=Simulink  SourceProductBaseCode=SL
  Bit Shift : Subsystem  TreatAsAtomicUnit=on  mask(Bit Shift){mode=Shift Left Logical, N=0}
      mask prompts: mode "Shift Mode"; N "Shift Length (must be greater than or equal to zero)"
      mask help: Perform a logical or arithmetic shift on the input signal, as specified by the Shift Mode parameter. The Shift Length specifies the number of bits shifted.
      mask init:
      | blkname = hdlblkmask_bitshift;
      mask Help: helpview([docroot '/simulink/helptargets.map'],'HDL_bit_shift');
      mask TypeOptions mode: Shift Left Logical | Shift Right Logical | Shift Right Arithmetic
      mask Display: disp(blkname);
  Bit Slice : Subsystem  TreatAsAtomicUnit=on  mask(Bit Slice){lidx=7, ridx=0}
      mask prompts: lidx "MSB Position"; ridx "LSB Position"
      mask help: Return a consecutive field of bits from the input signal. The field is indexed (0-based relative to LSB) by the LSB Position and MSB Position.
      mask init:
      | blkname = hdlblkmask_bitslice;
      mask Help: helpview([docroot '/simulink/helptargets.map'],'HDL_bit_slice');
      mask Display: disp(blkname);
  Bitwise Operator : simulink/Logic and Bit Operations/Bitwise Operator  logicop=AND  UseBitMask=on  BitMask=bin2dec('11011001')  BitMaskRealWorld=Stored Integer
  Compare To Constant : simulink/Logic and Bit Operations/Compare To Constant  relop=<=  const=3.0  OutDataTypeStr=boolean
  Compare To Zero : simulink/Logic and Bit Operations/Compare To Zero  relop=<=  OutDataTypeStr=boolean
  Detect Change : simulink/Logic and Bit Operations/Detect Change  vinit=0  OutDataTypeStr=boolean
  Detect Decrease : simulink/Logic and Bit Operations/Detect Decrease  vinit=0.0  OutDataTypeStr=boolean
  Detect Increase : simulink/Logic and Bit Operations/Detect Increase  vinit=0.0  OutDataTypeStr=boolean
  Extract Bits : simulink/Logic and Bit Operations/Extract Bits  bitsToExtract=Upper half  numBits=8  bitIdxRange=[0 7]  outScalingMode=Preserve fixed-point scaling
      settings: SourceProductName=Simulink
  Logical Operator : Logic  AllPortsSameDT=off  OutDataTypeStr=boolean
  Relational Operator : RelationalOperator  Operator=<=  OutDataTypeStr=boolean  RndMeth=Nearest
  Shift Arithmetic : ArithShift  BitShiftNumber=8

== system hdlsllibUNLOCKED/Lookup Tables ==
  1-D Lookup Table : Lookup_n-D  NumberOfTableDimensions=1  LookupTableObject=''  BreakpointsForDimension1=[-5:5]  BreakpointsForDimension1FirstPoint=10  BreakpointsForDimension2FirstPoint=10  BreakpointsForDimension1Spacing=12  BreakpointsForDimension2Spacing=12  IndexSearchMethod=Evenly spaced points  Table=tanh([-5:5])  InterpMethod=Flat  DiagnosticForOutOfRangeInput=Error  InternalRulePriority=Speed  RndMeth=Simplest  InputSameDT=on
  2-D Lookup Table : Lookup_n-D  LookupTableObject=''  BreakpointsForDimension1=[1:2]  BreakpointsForDimension2=[1:2]  BreakpointsForDimension1FirstPoint=10  BreakpointsForDimension2FirstPoint=10  BreakpointsForDimension1Spacing=12  BreakpointsForDimension2Spacing=12  IndexSearchMethod=Evenly spaced points  Table=[4 5;16 19]  InterpMethod=Flat  DiagnosticForOutOfRangeInput=Error  InternalRulePriority=Speed  RndMeth=Simplest  InputSameDT=on
  Cosine HDL Optimized : Subsystem  mask(Sine and Cosine HDL optimized block){OutputFormula=cos(2*pi*u), NumDataPoints=64, TableDataTypeStr=fixdt(0,16,15), SimulateLUTROMDelay=off}
      mask prompts: OutputFormula "Simulink:masks:OutputFormula_MP"; NumDataPoints "HDLShared:hdlshared:CosineHDL_Npts"; TableDataTypeStr "Simulink:blkprm_prompts:TABLE_UNIFIEDDATATYPE"; SimulateLUTROMDelay "HDLShared:hdlshared:CosineHDL_Map2RAM"
      mask help: Sine and Cosine HDL optimized block using quarter wave symmetry, and HDL friendly settings.
      mask init:
      | curr_blk_name=gcb;
      | sys_name=gcs;
      | 
      | hdlblkmask_sincos(curr_blk_name,sys_name,OutputFormula,...
      |     NumDataPoints,TableDataTypeStr,SimulateLUTROMDelay);
      | SampleTime=-1;
      mask Help: helpview([docroot '/simulink/helptargets.map'],'SineAndCosineHDL_Optimized');
      mask TypeOptions OutputFormula: sin(2*pi*u) | cos(2*pi*u) | exp(j*2*pi*u) | sin(2*pi*u) and cos(2*pi*u)
      mask DialogControl DescGroupVar Prompt: HDLShared:hdlshared:SineAndCosineHDL_Title
      mask DialogControl DetailedDescription Prompt: HDLShared:hdlshared:SineAndCosineHDL_Description
      mask DialogControl OutputFormula Prompt: Output formula
      mask DialogControl NumDataPoints Prompt: Number of data points
      mask DialogControl TableDataTypeStr Prompt: Table data type:
      mask DialogControl SimulateLUTROMDelay Prompt: Simulate RAM Delay
      mask Display:
      | port_label('input',1,'u')
      | port_label('output',1,'cos(2*pi*u)')
      | xpos = 0.35;
      | yoffset = 0.5;
      | if ( SimulateLUTROMDelay )
      |   text(xpos,yoffset,'HDL (Z^{-1})','texmode','on')
      | else
      |    text(xpos,yoffset,'HDL')
      | end
  Direct Lookup Table (n-D) : LookupNDDirect  Table=[4 5 ;16 19 ]  DiagnosticForOutOfRangeInput=Error
  Prelookup : PreLookup  BreakpointsData=[10:10:80]  IndexSearchMethod=Evenly spaced points  UseLastBreakpoint=on  DiagnosticForOutOfRangeInput=Error
  Sine HDL Optimized : $bdroot/Lookup Tables/Cosine HDL Optimized  OutputFormula=sin(2*pi*u)  NumDataPoints=64  TableDataTypeStr=fixdt(0,16,15)  SimulateLUTROMDelay=off
  n-D Lookup Table : Lookup_n-D  LookupTableObject=''  BreakpointsForDimension1=[1:2]  BreakpointsForDimension2=[1:2]  BreakpointsForDimension3=[5, 7]  BreakpointsForDimension1FirstPoint=10  BreakpointsForDimension2FirstPoint=10  BreakpointsForDimension1Spacing=12  BreakpointsForDimension2Spacing=12  IndexSearchMethod=Evenly spaced points  Table=[4 5;16 19]  InterpMethod=Flat  DiagnosticForOutOfRangeInput=Error  InternalRulePriority=Speed  RndMeth=Simplest  InputSameDT=on

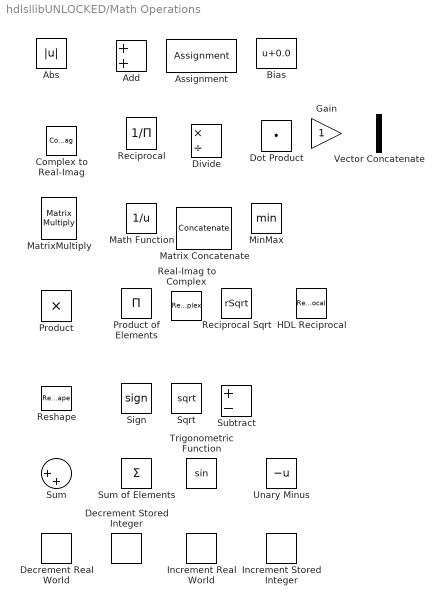
== system hdlsllibUNLOCKED/Math Operations ==
  Abs : Abs
  Add : Sum
  Assignment : Assignment  IndexOptions=Index vector (dialog)  Indices=1  OutputSizes=1
  Bias : Bias  Bias=0.0
  Complex to Real-Imag : ComplexToRealImag
  Decrement Real World : simulink/Additional Math & Discrete/Additional Math: Increment - Decrement/Decrement Real World
      settings: SourceProductName=Simulink  SourceProductBaseCode=SL
  Decrement Stored Integer : simulink/Additional Math & Discrete/Additional Math: Increment - Decrement/Decrement Stored Integer
      settings: SourceProductName=Simulink  SourceProductBaseCode=SL
  Divide : Product  Inputs=*/  SaturateOnIntegerOverflow=on  RndMeth=Zero
  Dot Product : DotProduct  InputSameDT=on  OutDataTypeStr=Inherit: Inherit via internal rule
  Gain : Gain
  HDL Reciprocal : Reciprocal
  Increment Real World : simulink/Additional Math & Discrete/Additional Math: Increment - Decrement/Increment Real World
      settings: SourceProductName=Simulink  SourceProductBaseCode=SL
  Increment Stored Integer : simulink/Additional Math & Discrete/Additional Math: Increment - Decrement/Increment Stored Integer
      settings: SourceProductName=Simulink
  Math Function : Math  Operator=reciprocal  RndMeth=Zero  SaturateOnIntegerOverflow=on
  Matrix Concatenate : Concatenate  Mode=Multidimensional array  ConcatenateDimension=2
  MatrixMultiply : Product  Multiplication=Matrix(*)
  MinMax : MinMax
  Product : Product
  Product of Elements : Product  Inputs=*
  Real-Imag to Complex : RealImagToComplex
  Reciprocal : Product  Inputs=/  SaturateOnIntegerOverflow=on  RndMeth=Zero
  Reciprocal Sqrt : Sqrt  Operator=rSqrt  AlgorithmType=Newton-Raphson  SaturateOnIntegerOverflow=on
  Reshape : Reshape
  Sign : Signum
  Sqrt : Sqrt  SaturateOnIntegerOverflow=on
  Subtract : Sum  Inputs=+-
  Sum : Sum  Inputs=|++
  Sum of Elements : Sum  Inputs=+
  Trigonometric Function : Trigonometry  ApproximationMethod=CORDIC
  Unary Minus : UnaryMinus
  Vector Concatenate : Concatenate

== system hdlsllibUNLOCKED/Model Verification ==
  Assertion : Assertion
  Check Discrete Gradient : simulink/Model Verification/Check Discrete Gradient  Description=| du / dt | < 1  gradient=1  enabled=on  stopWhenAssertionFail=on  export=off  icon=graphic
      settings: SourceProductName=Simulink  SourceProductBaseCode=SL
  Check Dynamic Gap : simulink/Model Verification/Check  Dynamic Gap  Description=u < min || max < u  enabled=on  stopWhenAssertionFail=on  export=off  icon=graphic
      settings: SourceProductName=Simulink  SourceProductBaseCode=SL
  Check Dynamic Range : simulink/Model Verification/Check  Dynamic Range  Description=min < u < max  enabled=on  stopWhenAssertionFail=on  export=off  icon=graphic
      settings: SourceProductName=Simulink  SourceProductBaseCode=SL
  Check Static Gap : simulink/Model Verification/Check  Static Gap  Description=u <= 0 || 100 <= u  max=100  max_included=on  min=0  min_included=on  enabled=on  stopWhenAssertionFail=on  export=off  icon=graphic
      settings: SourceProductName=Simulink  SourceProductBaseCode=SL
  Check Static Range : simulink/Model Verification/Check  Static Range  Description=0 <= u <= 100  max=100  max_included=on  min=0  min_included=on  enabled=on  stopWhenAssertionFail=on  export=off  icon=graphic
      settings: SourceProductName=Simulink  SourceProductBaseCode=SL
  Check Dynamic Lower Bound : simulink/Model Verification/Check Dynamic  Lower Bound  Description=min < u  Enabled=on  stopWhenAssertionFail=on  export=off  icon=graphic
      settings: SourceProductName=Simulink  SourceProductBaseCode=SL
  Check Dynamic Upper Bound : simulink/Model Verification/Check Dynamic  Upper Bound  Description=u < max  enabled=on  stopWhenAssertionFail=on  export=off  icon=graphic
      settings: SourceProductName=Simulink  SourceProductBaseCode=SL
  Check Input Resolution : simulink/Model Verification/Check Input  Resolution  Description=-Inf < u < +Inf  resolution=1  enabled=on  stopWhenAssertionFail=on  export=off
      settings: SourceProductName=Simulink  SourceProductBaseCode=SL
  Check Static Lower Bound : simulink/Model Verification/Check Static  Lower Bound  Description=0 <= u  min=0  min_included=on  enabled=on  stopWhenAssertionFail=on  export=off  icon=graphic
      settings: SourceProductName=Simulink
  Check Static Upper Bound : simulink/Model Verification/Check Static  Upper Bound  Description=u <= 0  max=0  max_included=on  enabled=on  stopWhenAssertionFail=on  export=off  icon=graphic
      settings: SourceProductName=Simulink  SourceProductBaseCode=SL

== system hdlsllibUNLOCKED/Model-Wide Utilities ==
  DocBlock : simulink/Model-Wide Utilities/DocBlock  DocumentType=Text
  Model Info : simulink/Model-Wide Utilities/Model Info  Frame=on  DisplayStringWithTags=Model Info  HorizontalTextAlignment=Center  LeftAlignmentValue=0.5

== system hdlsllibUNLOCKED/Ports & Subsystems ==
  In1 : Inport
  In Bus Element : Inport  Port=2  PortName=InBus  Element=signal1
  Enable : EnablePort
  Trigger : TriggerPort  VariantControl=Variant  PortDimensions=1
  Atomic Subsystem : simulink/Ports & Subsystems/Atomic Subsystem
      settings: SourceProductName=Simulink  SourceProductBaseCode=SL
  Enabled Subsystem : Subsystem  TreatAsAtomicUnit=on  mask(Enable Subsystem){}
      mask help: Simulink:masks:EnabledSubsystem_MD
      settings: CopyFcn=set_param(gcbh,'LinkStatus','breakWithoutHierarchy'); set_param(gcbh,'Mask','off'); set_param(gcbh,'MaskType',''); set_param(gcbh,'MaskDescription',''); set_param(gcbh,'OpenFcn',''); set_param(gcbh,'CopyFcn','')  OpenFcn=open_system(gcbh,'force')
  For Each Subsystem : simulink/Ports & Subsystems/For Each Subsystem
      settings: SourceProductName=Simulink  SourceProductBaseCode=SL
  Model : ModelReference  SimulationMode=Normal
  Subsystem : simulink/Ports & Subsystems/Subsystem
      settings: SourceProductName=Simulink  SourceProductBaseCode=SL
  Triggered Subsystem : simulink/Ports & Subsystems/Triggered Subsystem
      settings: SourceProductName=Simulink  SourceProductBaseCode=SL
  Variant Subsystem : simulink/Ports & Subsystems/Variant Subsystem
      settings: SourceProductName=Simulink  SourceProductBaseCode=SL
  Out1 : Outport
  Out Bus Element : Outport  Port=2  PortName=OutBus  Element=signal1

== system hdlsllibUNLOCKED/Signal Attributes ==
  Bus to Vector : BusToVector
  Data Type Duplicate : DataTypeDuplicate
  Data Type Propagation : simulink/Signal Attributes/Data Type Propagation  PropDataType=fixdt(1, 16)  IfRefDouble=double  IfRefSingle=single  IsSigned=IsSigned1 or IsSigned2  NumBitsBase=max([NumBits1 NumBits2])  NumBitsMult=1  NumBitsAdd=0  NumBitsAllowFinal=1:128  PropScaling=2^-10  ValuesUsedBestPrec=[5 -7]  SlopeBase=min([Slope1 Slope2])  SlopeMult=1  SlopeAdd=0  BiasBase=Bias1  BiasMult=1  BiasAdd=0
      settings: SourceProductName=Simulink  SourceProductBaseCode=SL
  Data Type Conversion : DataTypeConversion
  Probe : Probe  ProbeSignalDimensions=on  ProbeWidthDataType=Same as input  ProbeSampleTimeDataType=Same as input  ProbeComplexityDataType=Same as input  ProbeDimensionsDataType=Same as input
  Rate Transition : RateTransition
  Signal Conversion : SignalConversion  OverrideOpt=off
  Signal Specification : SignalSpecification

== system hdlsllibUNLOCKED/Signal Routing ==
  Bus Element In : Inport  PortName=InBus  Element=signal1
  Bus Assignment : BusAssignment  AssignedSignals=signal1
  Bus Creator : BusCreator  Inputs=2
  Bus Selector : BusSelector  OutputSignals=signal1,signal2
  Demux : Demux  Outputs=2
  Index Vector : MultiPortSwitch  DataPortOrder=Zero-based contiguous  Inputs=1  zeroidx=on
  Multiport Switch : MultiPortSwitch
  Mux : Mux  Inputs=2
  Selector : Selector  InputPortWidth=3  IndexOptions=Index vector (dialog)  Indices=[1 3]  OutputSizes=1
  Switch : Switch
  Vector Concatenate : Concatenate
  Bus Element Out : Outport  PortName=OutBus  Element=signal1

== system hdlsllibUNLOCKED/Sinks ==
  Display : Display
  Floating Scope : Scope
      settings: Floating=on
  Scope : Scope
  Stop Simulation : Stop
  Terminator : Terminator
  To File : ToFile  SaveFormat=Timeseries
  To Workspace : ToWorkspace  VariableName=simout  SaveFormat=Timeseries  SampleTime=-1
  XY Graph : simulink/Sinks/XY Graph  xmin=-1  xmax=1  ymin=-1  ymax=1  st=-1
  Out1 : Outport
  Out Bus Element : Outport  Port=2  PortName=OutBus  Element=signal1

== system hdlsllibUNLOCKED/Sources ==
  In1 : Inport
  In Bus Element : Inport  Port=2  PortName=InBus  Element=signal1
  Constant : Constant  SampleTime=-1
  Counter Free-Running : simulink/Sources/Counter Free-Running  NumBits=16  tsamp=-1
  Counter Limited : simulink/Sources/Counter Limited  uplimit=7  tsamp=-1
  Enumerated Constant : simulink/Sources/Enumerated Constant  OutDataTypeStr=Enum: HDLStatusEnum  Value=HDLStatusEnum.Ready  SampleTime=-1
      settings: SourceProductName=Simulink
  Ground : Ground
  HDL Counter : Subsystem  mask(HDL Counter){CountType=Count limited, CountInit=0, CountStep=1, CountMax=25, CountFromType=Initial value, CountFrom=0, CountResetPort=off, CountLoadPort=off, CountEnbPort=off, CountDirPort=off, CountDataType=Unsigned, CountWordLen=8, CountFracLen=0, CountSampTime=1}
      mask prompts: CountType "Counter type:"; CountInit "Initial value:"; CountStep "Step value:"; CountMax "Count to value:"; CountFromType "Count from:"; CountFrom "Count from value:"; CountResetPort "Local reset port"; CountLoadPort "Load ports"; CountEnbPort "Count enable port"; CountDirPort "Count direction port"; CountDataType "Counter output data is:"; CountWordLen "Word length:"; CountFracLen "Fraction length:"; CountSampTime "Sample time:"
      mask help: Counter for HDL code generation.
      mask init:
      | issigned = double(strcmp(get_param(gcb, 'CountDataType'), 'Signed'));
      | [maxval_sc freerun samptime] = hdlblkmask_counter;
      mask Help: helpview([docroot '/simulink/helptargets.map'],'HDL_Counter');
      mask TypeOptions CountType: Free running | Count limited
      mask Callback CountType: hdlblkmask_counter
      mask Callback CountInit: hdlblkmask_counter
      mask TypeOptions CountFromType: Initial value | Specify
      mask Callback CountFromType: hdlblkmask_counter
      mask Callback CountResetPort: hdlblkmask_counter
      mask Callback CountLoadPort: hdlblkmask_counter
      mask Callback CountEnbPort: hdlblkmask_counter
      mask Callback CountDirPort: hdlblkmask_counter
      mask TypeOptions CountDataType: Unsigned | Signed

== system hdlsllibUNLOCKED/User-Defined Functions ==
  MATLAB Function : MATLAB Function  TreatAsAtomicUnit=on
  MATLAB System : MATLABSystem

== system hdlsllibUNLOCKED/Discrete/Unit Delay Enabled Synchronous ==
  u : Inport
  E : Inport  Port=2
  Unit Delay Enabled : Subsystem
  y : Outport
  wires:
  u/1 -> Unit Delay Enabled/1(u)
  E/1 -> Unit Delay Enabled/2(E)
  Unit Delay Enabled/1(y) -> y/1
